simulink model "Complete_scheme_Prove_Balancing"  (R2021a)
settings: Solver=VariableStepAuto  StartTime=0.0  StopTime=60  RelTol=1e-8
PreLoadFcn:
  | data_preload
  | input_preload
values from neighbouring files (symbols this model uses):
  A = [-1/sqrt(2)  1/sqrt(2)     0;      -1/sqrt(6) -1/sqrt(6) sqrt(2/3);       1/sqrt(3)  1/sqrt(3) 1/sqrt(3)]    [data_preload.m]    (also in data_preload_4RW.m = [-a  a  a -a;      -a -a  a  a;       a  a  a  a])
  A_inv = pinv(A)    [data_preload.m]    (also in data_preload_4RW.m)
  A_rw = [-b/J*eye(3) Kt/J*eye(3); -Ke/L*eye(3) -R/L*eye(3)]    [data_preload.m]    (also in data_preload_4RW.m = [-b/J*eye(4) Kt/J*eye(4); -Ke/L*eye(4) -R/L*eye(4)])
  B_rw = [zeros(3); 1/L*eye(3)]    [data_preload.m]    (also in data_preload_4RW.m = [zeros(4); 1/L*eye(4)])
  C_rw = [eye(6); -b/J*eye(3) Kt/J*eye(3)]    [data_preload.m]    (also in data_preload_4RW.m = [eye(8); -b/J*eye(4) Kt/J*eye(4)])
  dt = 0.00001    (= 1e-05)    [RWSizing.m]    (also in data_preload.m = 0.01; data_preload_4RW.m = 0.01)
  G_aug = lqr(A_aug,B_aug,Qlqr,Rlqr)    [data_preload.m]    (also in data_preload_4RW.m)
  G_sim = lqr(A_sim,B_sim,Qlqr,Rlqr)    [data_preload.m]    (also in data_preload_4RW.m)
  I_s = [0.107 0 0; 0 0.108 0; 0 0 0.116]    [data_preload.m]    (also in data_preload_4RW.m)
  I_s_inv = inv(I_s)    [data_preload.m]    (also in data_preload_4RW.m)
  I_w = J*eye(3)    [data_preload.m]    (also in data_preload_4RW.m = J*eye(4))
  I_w_inv = inv(I_w)    [data_preload.m]    (also in data_preload_4RW.m)
  J = 1.74e-4 + 5.1e-7    (= 0.00017451)    [data_preload.m]    (also in data_preload_4RW.m)
  Ke = 0.008    [data_preload.m]    (also in data_preload_4RW.m)
  Kt = 0.00797    [data_preload.m]    (also in data_preload_4RW.m)
  omega = omega*2*pi/60    (= 188.495559215)    [RWSizing.m]    (also in data_preload.m = 250; data_preload_4RW.m = 250)
  vel_slope = theta_tot/(n*t_tot^2*(1-n))    (= 0.0517844942899)    [input_preload.m]
undefined symbols (not defined in the file or in its folder): DiscIntNeverNeededParam
libraries: simulink x28, simulink_extras x14, vrlib x7
settings Model: Creator=gcors  LastModifiedBy=gcors
settings DataIOCC: SaveFormat=Structure

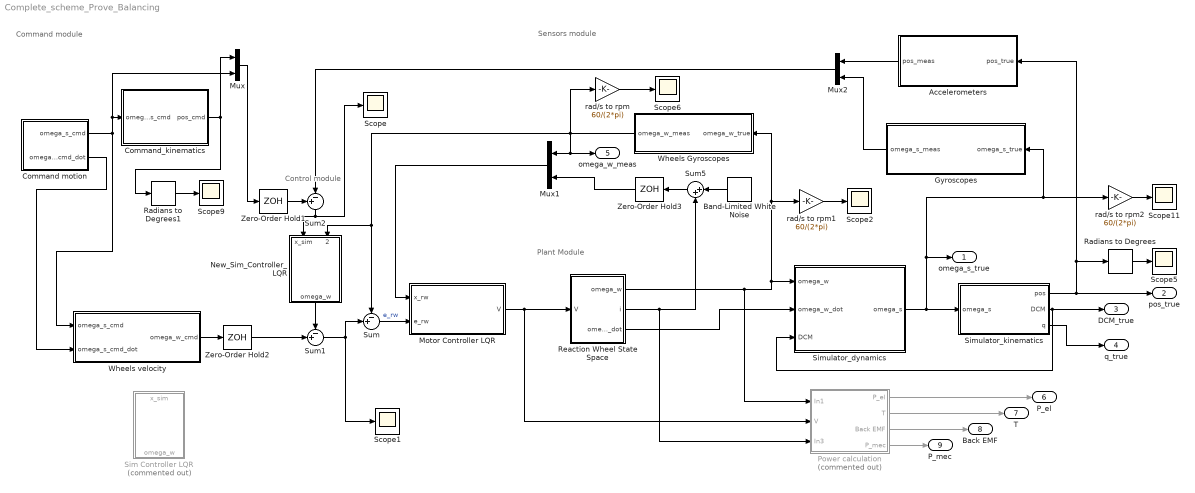
== system Complete_scheme_Prove_Balancing ==
  note: Control module
  note: Sensors module
  note: Plant Module
  note: Command module
  Accelerometers : Subsystem
  Band-Limited White Noise : simulink/Sources/Band-Limited White Noise  Cov=[(0.1^2)/47]  Ts=dt  seed=[23341]
  Command motion : Subsystem
  Command_kinematics : Subsystem
  Gyroscopes : Subsystem
  Motor Controller LQR : Subsystem
  Mux : Mux  Inputs=2
  Mux1 : Mux  Inputs=2
  Mux2 : Mux  Inputs=2
  New_Sim_Controller_LQR : Subsystem
  Power calculation : Subsystem  Commented=on
  Radians to Degrees : simulink_extras/Transformations/Radians to Degrees
  Radians to Degrees1 : simulink_extras/Transformations/Radians to Degrees
  Reaction Wheel State Space : Subsystem
  Scope{,1..2,5..6,9,11} (7 alike) : Scope
  Sim Controller LQR : Subsystem  Commented=on
  Simulator_dynamics : Subsystem
  Simulator_kinematics : Subsystem
  Sum : Sum  Inputs=-+|
  Sum1 : Sum  Inputs=-+|
  Sum2 : Sum  Inputs=+-|
  Sum5 : Sum  Inputs=|++
  Wheels Gyroscopes : Subsystem
  Wheels velocity : Subsystem
  Zero-Order Hold1 : ZeroOrderHold  SampleTime=dt
  Zero-Order Hold2 : ZeroOrderHold  SampleTime=dt
  Zero-Order Hold3 : ZeroOrderHold  SampleTime=dt
  rad/s to rpm : Gain  Gain=60/(2*pi)
  rad/s to rpm1 : Gain  Gain=60/(2*pi)
  rad/s to rpm2 : Gain  Gain=60/(2*pi)
  omega_s_true : Outport  PortDimensions=3
  pos_true : Outport  Port=2  PortDimensions=3
  DCM_true : Outport  Port=3  PortDimensions=[3,3]
  q_true : Outport  Port=4
  omega_w_meas : Outport  Port=5  PortDimensions=3
  P_el : Outport  Port=6
  T : Outport  Port=7
  Back EMF : Outport  Port=8
  P_mec : Outport  Port=9
  wires:
  Simulator_dynamics/1(omega_s) -> rad/s to rpm2/1, Gyroscopes/1(omega_s_true), omega_s_true/1, Simulator_kinematics/1(omega_s)
  Sum/1 -> Motor Controller LQR/2(e_rw)  "e_rw"
  Simulator_kinematics/3(q) -> q_true/1
  Simulator_kinematics/2(DCM) -> Simulator_dynamics/3(DCM), DCM_true/1
  Reaction Wheel State Space/3(omega_w_dot) -> Simulator_dynamics/2(omega_w_dot)
  Radians to Degrees1/1 -> Scope9/1
  Command_kinematics/1(pos_cmd) -> Mux/1, Radians to Degrees1/1
  Command motion/1(omega_s_cmd) -> Mux/2, Command_kinematics/1(omega_s_cmd), Wheels velocity/1(omega_s_cmd)
  Command motion/2(omega_s_cmd_dot) -> Wheels velocity/2(omega_s_cmd_dot)
  Sum1/1 -> Scope1/1, Sum/2
  rad/s to rpm/1 -> Scope6/1
  Reaction Wheel State Space/2(i) -> Sum5/2, Power calculation/3(In3)
  Simulator_kinematics/1(pos) -> Accelerometers/1(pos_true), Radians to Degrees/1, pos_true/1
  Gyroscopes/1(omega_s_meas) -> Mux2/2
  Accelerometers/1(pos_meas) -> Mux2/1
  Mux2/1 -> Sum2/2
  Band-Limited White Noise/1 -> Sum5/1
  Power calculation/1(P_el) -> P_el/1
  Power calculation/2(T) -> T/1
  Power calculation/3(Back EMF) -> Back EMF/1
  Power calculation/4(P_mec) -> P_mec/1
  Mux1/1 -> Motor Controller LQR/1(x_rw)
  Wheels velocity/1(omega_w_cmd) -> Zero-Order Hold2/1
  Mux/1 -> Zero-Order Hold1/1
  Radians to Degrees/1 -> Scope5/1
  Reaction Wheel State Space/1(omega_w) -> Simulator_dynamics/1(omega_w), Wheels Gyroscopes/1(omega_w_true), rad/s to rpm1/1, Power calculation/1(In1)
  Wheels Gyroscopes/1(omega_w_meas) -> rad/s to rpm/1, New_Sim_Controller_LQR/2(omega_w_meas), Sum/1, omega_w_meas/1, Mux1/1
  rad/s to rpm1/1 -> Scope2/1
  Motor Controller LQR/1(V) -> Reaction Wheel State Space/1(V), Power calculation/2(V)
  rad/s to rpm2/1 -> Scope11/1
  Sum5/1 -> Zero-Order Hold3/1
  Zero-Order Hold2/1 -> Sum1/2
  Zero-Order Hold3/1 -> Mux1/2
  Zero-Order Hold1/1 -> Sum2/1
  Sum2/1 -> New_Sim_Controller_LQR/1(x_sim), Scope/1
  New_Sim_Controller_LQR/1(omega_w) -> Sum1/1

== system Complete_scheme_Prove_Balancing/Accelerometers ==
  pos_true : Inport
  Accelerometers model x1 : Subsystem
  Accelerometers model x2 : Subsystem
  Accelerometers model x3 : Subsystem
  Demux2 : Demux  Outputs=3
  Manual Switch : ManualSwitch  CurrentSetting=0
  Mux1 : Mux  Inputs=3
  Zero-Order Hold : ZeroOrderHold  SampleTime=dt
  pos_meas : Outport
  wires:
  Accelerometers model x1/1(pos_xmeas) -> Mux1/1
  Demux2/1 -> Accelerometers model x1/1(pos_x)
  Accelerometers model x2/1(pos_xmeas) -> Mux1/2
  Demux2/2 -> Accelerometers model x2/1(pos_x)
  pos_true/1 -> Manual Switch/1, Demux2/1
  Demux2/3 -> Accelerometers model x3/1(pos_x)
  Accelerometers model x3/1(pos_xmeas) -> Mux1/3
  Mux1/1 -> Manual Switch/2
  Manual Switch/1 -> Zero-Order Hold/1
  Zero-Order Hold/1 -> pos_meas/1

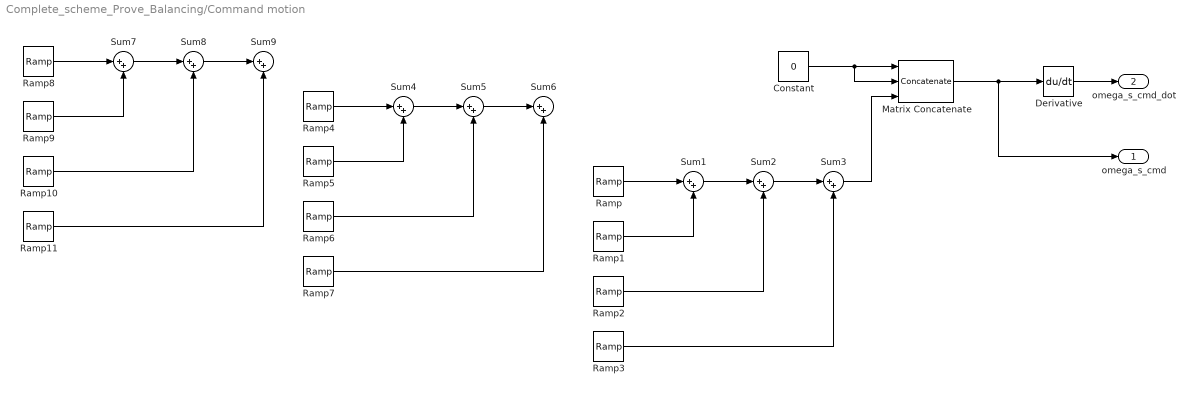
== system Complete_scheme_Prove_Balancing/Command motion ==
  Constant : Constant  Value=0
  Derivative : Derivative
  Matrix Concatenate : Concatenate  NumInputs=3  ConcatenateDimension=2
  Ramp : simulink/Sources/Ramp  slope=vel_slope  start=t0  InitialOutput=0
  Ramp1 : simulink/Sources/Ramp  slope=-vel_slope  start=t1  InitialOutput=0
  Ramp10 : simulink/Sources/Ramp  slope=-0.03  start=52  InitialOutput=0
  Ramp11 : simulink/Sources/Ramp  slope=0.03  start=55  InitialOutput=0
  Ramp2 : simulink/Sources/Ramp  slope=-vel_slope  start=t2  InitialOutput=0
  Ramp3 : simulink/Sources/Ramp  slope=vel_slope  start=t3  InitialOutput=0
  Ramp4 : simulink/Sources/Ramp  slope=0.05  start=30  InitialOutput=0
  Ramp5 : simulink/Sources/Ramp  slope=-0.05  start=33  InitialOutput=0
  Ramp6 : simulink/Sources/Ramp  slope=-0.05  start=37  InitialOutput=0
  Ramp7 : simulink/Sources/Ramp  slope=0.05  start=40  InitialOutput=0
  Ramp8 : simulink/Sources/Ramp  slope=0.03  start=45  InitialOutput=0
  Ramp9 : simulink/Sources/Ramp  slope=-0.03  start=48  InitialOutput=0
  Sum{1..9} (9 alike) : Sum  Inputs=|++
  omega_s_cmd : Outport
  omega_s_cmd_dot : Outport  Port=2
  wires:
  Sum2/1 -> Sum3/1
  Ramp3/1 -> Sum3/2
  Ramp/1 -> Sum1/1
  Ramp1/1 -> Sum1/2
  Ramp2/1 -> Sum2/2
  Sum1/1 -> Sum2/1
  Derivative/1 -> omega_s_cmd_dot/1
  Matrix Concatenate/1 -> Derivative/1, omega_s_cmd/1
  Sum4/1 -> Sum5/1
  Ramp7/1 -> Sum6/2
  Ramp5/1 -> Sum4/2
  Ramp4/1 -> Sum4/1
  Ramp6/1 -> Sum5/2
  Sum5/1 -> Sum6/1
  Sum7/1 -> Sum8/1
  Ramp11/1 -> Sum9/2
  Ramp9/1 -> Sum7/2
  Ramp8/1 -> Sum7/1
  Ramp10/1 -> Sum8/2
  Sum8/1 -> Sum9/1
  Constant/1 -> Matrix Concatenate/1, Matrix Concatenate/2
  Sum3/1 -> Matrix Concatenate/3

== system Complete_scheme_Prove_Balancing/Command_kinematics ==
  omega_s_cmd : Inport  PortDimensions=3
  Euler_angles : MATLAB Function  TreatAsAtomicUnit=on
  Gain : Gain  Gain=1/2
  Integrator1 : Integrator  InitialCondition=[0 0 0 1]'
  Matrix Multiply4 : Product  Multiplication=Matrix(*)
  Normalize Vector : vrlib/Utilities/Normalize Vector  maxzero=0
  OMEGA_matrix : MATLAB Function  TreatAsAtomicUnit=on
  Scope : Scope
  Scope1 : Scope
  getDCM : MATLAB Function  TreatAsAtomicUnit=on
  pos_cmd : Outport  PortDimensions=3
  wires:
  Integrator1/1 -> Normalize Vector/1  "q"
  OMEGA_matrix/1(OMEGA) -> Matrix Multiply4/1
  Gain/1 -> Integrator1/1  "q_dot"
  Matrix Multiply4/1 -> Gain/1
  omega_s_cmd/1 -> OMEGA_matrix/1(omega_s)
  Normalize Vector/1 -> Euler_angles/1(q), Scope/1, Matrix Multiply4/2, getDCM/1(q)
  Euler_angles/1(pos) -> pos_cmd/1
  getDCM/1(DCM) -> Scope1/1

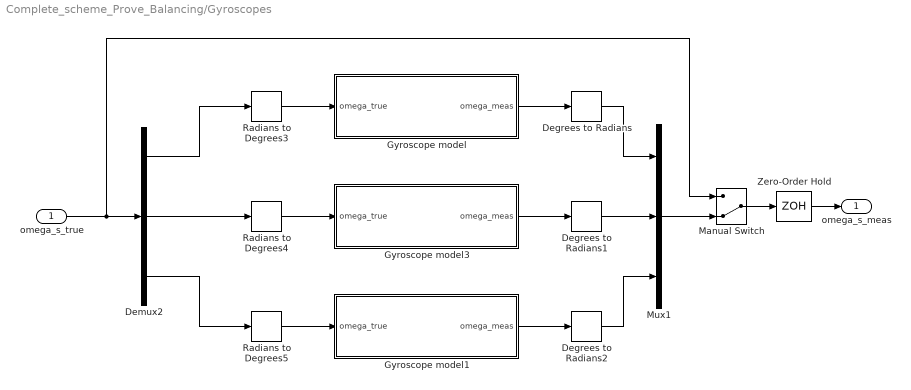
== system Complete_scheme_Prove_Balancing/Gyroscopes ==
  omega_s_true : Inport
  Degrees to Radians : simulink_extras/Transformations/Degrees to Radians
  Degrees to Radians1 : simulink_extras/Transformations/Degrees to Radians
  Degrees to Radians2 : simulink_extras/Transformations/Degrees to Radians
  Demux2 : Demux  Outputs=3
  Gyroscope model : Subsystem
  Gyroscope model1 : Subsystem
  Gyroscope model3 : Subsystem
  Manual Switch : ManualSwitch  CurrentSetting=0
  Mux1 : Mux  Inputs=3
  Radians to Degrees3 : simulink_extras/Transformations/Radians to Degrees
  Radians to Degrees4 : simulink_extras/Transformations/Radians to Degrees
  Radians to Degrees5 : simulink_extras/Transformations/Radians to Degrees
  Zero-Order Hold : ZeroOrderHold  SampleTime=dt
  omega_s_meas : Outport
  wires:
  Gyroscope model3/1(omega_meas) -> Degrees to Radians1/1
  Demux2/2 -> Radians to Degrees4/1
  Degrees to Radians/1 -> Mux1/1
  Demux2/1 -> Radians to Degrees3/1
  Gyroscope model/1(omega_meas) -> Degrees to Radians/1
  Demux2/3 -> Radians to Degrees5/1
  Degrees to Radians1/1 -> Mux1/2
  Radians to Degrees4/1 -> Gyroscope model3/1(omega_true)
  Degrees to Radians2/1 -> Mux1/3
  Radians to Degrees3/1 -> Gyroscope model/1(omega_true)
  Radians to Degrees5/1 -> Gyroscope model1/1(omega_true)
  Gyroscope model1/1(omega_meas) -> Degrees to Radians2/1
  omega_s_true/1 -> Demux2/1, Manual Switch/1
  Mux1/1 -> Manual Switch/2
  Manual Switch/1 -> Zero-Order Hold/1
  Zero-Order Hold/1 -> omega_s_meas/1

== system Complete_scheme_Prove_Balancing/Motor Controller LQR ==
  x_rw : Inport
  e_rw : Inport  Port=2  PortDimensions=3
  Discrete-Time Integrator : DiscreteIntegrator  gainval=1  SampleTime=-1  ICPrevOutput=DiscIntNeverNeededParam  ICPrevScaledInput=DiscIntNeverNeededParam
  G_aug : Constant  Value=G_aug
  Gain : Gain  Gain=-1
  Matrix Multiply : Product  Multiplication=Matrix(*)
  Mux : Mux  Inputs=2
  V : Outport
  wires:
  x_rw/1 -> Mux/1
  Mux/1 -> Matrix Multiply/2
  G_aug/1 -> Matrix Multiply/1
  Matrix Multiply/1 -> Gain/1
  Discrete-Time Integrator/1 -> Mux/2  "x_i"
  Gain/1 -> V/1
  e_rw/1 -> Discrete-Time Integrator/1

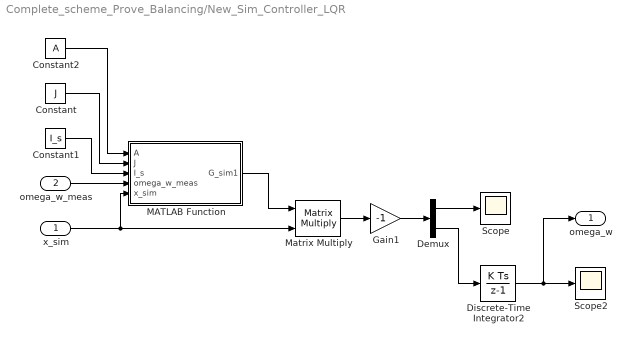
== system Complete_scheme_Prove_Balancing/New_Sim_Controller_LQR ==
  x_sim : Inport
  omega_w_meas : Inport  Port=2
  Constant : Constant  Value=J
  Constant1 : Constant  Value=I_s
  Constant2 : Constant  Value=A
  Demux : Demux  Outputs=2
  Discrete-Time Integrator2 : DiscreteIntegrator  gainval=1  SampleTime=dt  ICPrevOutput=DiscIntNeverNeededParam  ICPrevScaledInput=DiscIntNeverNeededParam
  Gain1 : Gain  Gain=-1
  MATLAB Function : MATLAB Function  TreatAsAtomicUnit=on  SystemSampleTime=dt*10
  Matrix Multiply : Product  Multiplication=Matrix(*)
  Scope : Scope
  Scope2 : Scope
  omega_w : Outport
  wires:
  Matrix Multiply/1 -> Gain1/1
  x_sim/1 -> MATLAB Function/5(x_sim), Matrix Multiply/2
  omega_w_meas/1 -> MATLAB Function/4(omega_w_meas)
  MATLAB Function/1(G_sim1) -> Matrix Multiply/1
  Constant/1 -> MATLAB Function/2(J)
  Constant1/1 -> MATLAB Function/3(I_s)
  Constant2/1 -> MATLAB Function/1(A)
  Discrete-Time Integrator2/1 -> omega_w/1, Scope2/1
  Gain1/1 -> Demux/1
  Demux/2 -> Discrete-Time Integrator2/1
  Demux/1 -> Scope/1

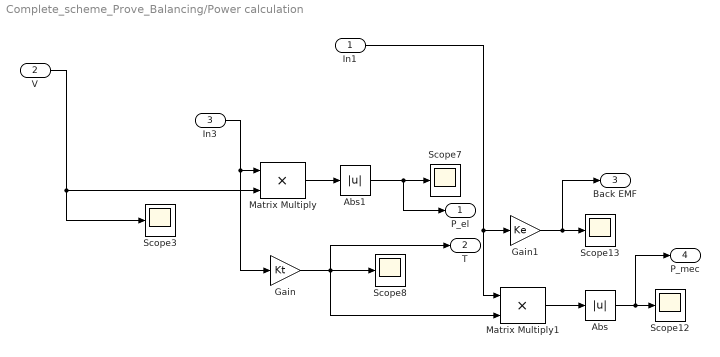
== system Complete_scheme_Prove_Balancing/Power calculation ==
  In1 : Inport
  V : Inport  Port=2
  In3 : Inport  Port=3
  Abs : Abs
  Abs1 : Abs
  Gain : Gain  Gain=Kt
  Gain1 : Gain  Gain=Ke
  Matrix Multiply : Product
  Matrix Multiply1 : Product
  Scope{3,7..8,12..13} (5 alike) : Scope
  P_el : Outport
  T : Outport  Port=2
  Back EMF : Outport  Port=3
  P_mec : Outport  Port=4
  wires:
  Gain/1 -> T/1, Scope8/1, Matrix Multiply1/2
  Matrix Multiply1/1 -> Abs/1
  In1/1 -> Gain1/1, Matrix Multiply1/1
  V/1 -> Matrix Multiply/2, Scope3/1
  Matrix Multiply/1 -> Abs1/1
  Gain1/1 -> Back EMF/1, Scope13/1
  Abs1/1 -> P_el/1, Scope7/1
  Abs/1 -> P_mec/1, Scope12/1
  In3/1 -> Gain/1, Matrix Multiply/1

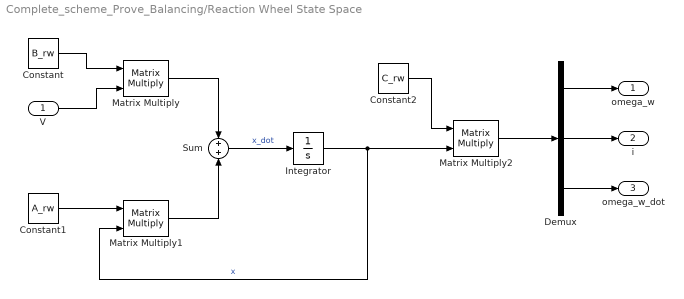
== system Complete_scheme_Prove_Balancing/Reaction Wheel State Space ==
  V : Inport  PortDimensions=3
  Constant : Constant  Value=B_rw
  Constant1 : Constant  Value=A_rw
  Constant2 : Constant  Value=C_rw
  Demux : Demux  Outputs=3
  Integrator : Integrator
  Matrix Multiply : Product  Multiplication=Matrix(*)
  Matrix Multiply1 : Product  Multiplication=Matrix(*)
  Matrix Multiply2 : Product  Multiplication=Matrix(*)
  Sum : Sum  Inputs=+|+
  omega_w : Outport  PortDimensions=3
  i : Outport  Port=2  PortDimensions=3
  omega_w_dot : Outport  Port=3
  wires:
  Integrator/1 -> Matrix Multiply2/2, Matrix Multiply1/2  "x"
  Constant1/1 -> Matrix Multiply1/1
  Matrix Multiply1/1 -> Sum/2
  Constant/1 -> Matrix Multiply/1
  Matrix Multiply/1 -> Sum/1
  Constant2/1 -> Matrix Multiply2/1
  Sum/1 -> Integrator/1  "x_dot"
  Matrix Multiply2/1 -> Demux/1
  Demux/3 -> omega_w_dot/1
  Demux/1 -> omega_w/1
  Demux/2 -> i/1
  V/1 -> Matrix Multiply/2

== system Complete_scheme_Prove_Balancing/Sim Controller LQR ==
  x_sim : Inport
  Discrete-Time Integrator1 : DiscreteIntegrator  gainval=1  SampleTime=dt  ICPrevOutput=DiscIntNeverNeededParam  ICPrevScaledInput=DiscIntNeverNeededParam
  G_sim : Constant  Value=G_sim
  Gain1 : Gain  Gain=-1
  Matrix Multiply : Product  Multiplication=Matrix(*)
  Scope : Scope
  Scope1 : Scope
  omega_w : Outport
  wires:
  G_sim/1 -> Matrix Multiply/1
  Matrix Multiply/1 -> Gain1/1
  x_sim/1 -> Matrix Multiply/2
  Gain1/1 -> Scope/1, Discrete-Time Integrator1/1
  Discrete-Time Integrator1/1 -> Scope1/1, omega_w/1

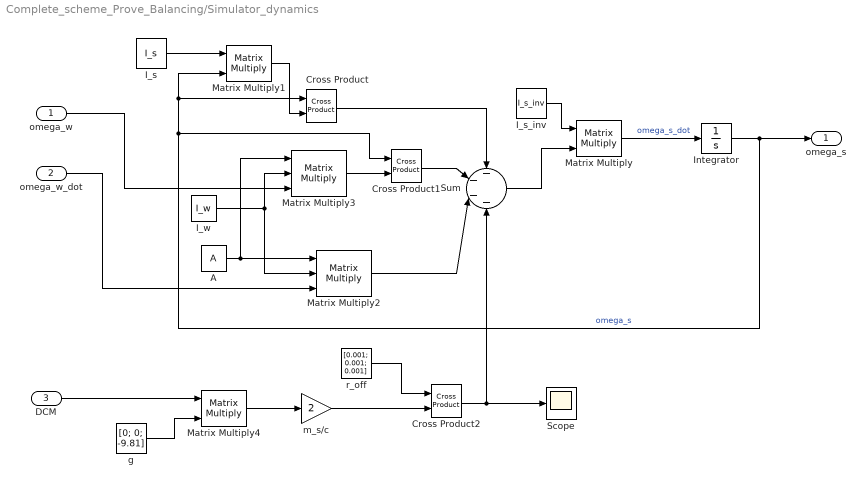
== system Complete_scheme_Prove_Balancing/Simulator_dynamics ==
  omega_w : Inport  PortDimensions=3
  omega_w_dot : Inport  Port=2  PortDimensions=3
  DCM : Inport  Port=3
  A : Constant  Value=A
  Cross Product : vrlib/Utilities/Cross Product
  Cross Product1 : vrlib/Utilities/Cross Product
  Cross Product2 : vrlib/Utilities/Cross Product
  I_s : Constant  Value=I_s
  I_s_inv : Constant  Value=I_s_inv
  I_w : Constant  Value=I_w
  Integrator : Integrator  InitialCondition=[0 0 0]'
  Matrix Multiply : Product  Multiplication=Matrix(*)
  Matrix Multiply1 : Product  Multiplication=Matrix(*)
  Matrix Multiply2 : Product  Inputs=3  Multiplication=Matrix(*)
  Matrix Multiply3 : Product  Inputs=3  Multiplication=Matrix(*)
  Matrix Multiply4 : Product  Multiplication=Matrix(*)
  Scope : Scope
  Sum : Sum  Inputs=----
  g : Constant  Value=[0; 0; -9.81]
  m_s/c : Gain  Gain=2
  r_off : Constant  Value=[0.001; 0.001; 0.001]
  omega_s : Outport  PortDimensions=3
  wires:
  Integrator/1 -> omega_s/1, Cross Product1/1, Cross Product/1, Matrix Multiply1/2  "omega_s"
  Matrix Multiply2/1 -> Sum/3
  I_w/1 -> Matrix Multiply3/2, Matrix Multiply2/2
  A/1 -> Matrix Multiply3/1, Matrix Multiply2/1
  Matrix Multiply3/1 -> Cross Product1/2
  I_s/1 -> Matrix Multiply1/1
  Matrix Multiply/1 -> Integrator/1  "omega_s_dot"
  Sum/1 -> Matrix Multiply/2
  Matrix Multiply1/1 -> Cross Product/2
  Cross Product/1 -> Sum/1
  omega_w/1 -> Matrix Multiply3/3
  Cross Product1/1 -> Sum/2
  omega_w_dot/1 -> Matrix Multiply2/3
  I_s_inv/1 -> Matrix Multiply/1
  DCM/1 -> Matrix Multiply4/1
  g/1 -> Matrix Multiply4/2
  Matrix Multiply4/1 -> m_s/c/1
  m_s/c/1 -> Cross Product2/2
  r_off/1 -> Cross Product2/1
  Cross Product2/1 -> Sum/4, Scope/1

== system Complete_scheme_Prove_Balancing/Simulator_kinematics ==
  omega_s : Inport  PortDimensions=3
  Euler_angles : MATLAB Function  TreatAsAtomicUnit=on
  Gain : Gain  Gain=1/2
  Integrator1 : Integrator  InitialCondition=[0 0 0 1]'
  Matrix Multiply4 : Product  Multiplication=Matrix(*)
  Normalize Vector : vrlib/Utilities/Normalize Vector  maxzero=0
  OMEGA_matrix : MATLAB Function  TreatAsAtomicUnit=on
  getDCM : MATLAB Function  TreatAsAtomicUnit=on
  pos : Outport  PortDimensions=3
  DCM : Outport  Port=2  PortDimensions=[3,3]
  q : Outport  Port=3  PortDimensions=4
  wires:
  Integrator1/1 -> Normalize Vector/1  "q"
  OMEGA_matrix/1(OMEGA) -> Matrix Multiply4/1
  Gain/1 -> Integrator1/1  "q_dot"
  Matrix Multiply4/1 -> Gain/1
  getDCM/1(DCM) -> DCM/1
  omega_s/1 -> OMEGA_matrix/1(omega_s)
  Normalize Vector/1 -> Euler_angles/1(q), q/1, Matrix Multiply4/2, getDCM/1(q)
  Euler_angles/1(pos) -> pos/1

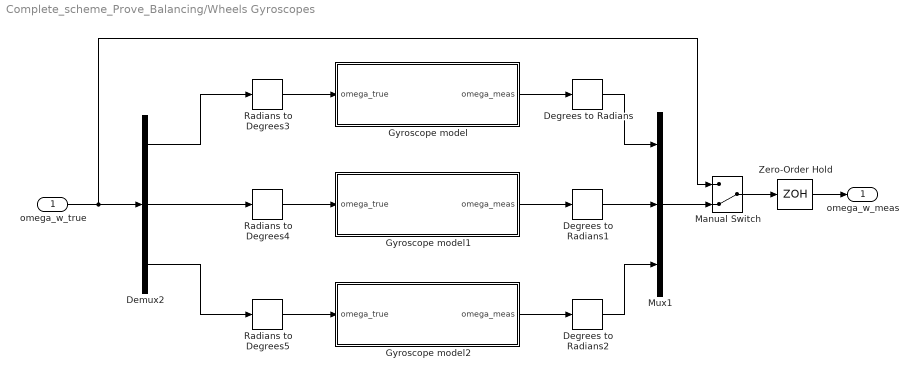
== system Complete_scheme_Prove_Balancing/Wheels Gyroscopes ==
  omega_w_true : Inport
  Degrees to Radians : simulink_extras/Transformations/Degrees to Radians
  Degrees to Radians1 : simulink_extras/Transformations/Degrees to Radians
  Degrees to Radians2 : simulink_extras/Transformations/Degrees to Radians
  Demux2 : Demux  Outputs=3
  Gyroscope model : Subsystem
  Gyroscope model1 : Subsystem
  Gyroscope model2 : Subsystem
  Manual Switch : ManualSwitch  CurrentSetting=0
  Mux1 : Mux  Inputs=3
  Radians to Degrees3 : simulink_extras/Transformations/Radians to Degrees
  Radians to Degrees4 : simulink_extras/Transformations/Radians to Degrees
  Radians to Degrees5 : simulink_extras/Transformations/Radians to Degrees
  Zero-Order Hold : ZeroOrderHold  SampleTime=dt
  omega_w_meas : Outport
  wires:
  Gyroscope model1/1(omega_meas) -> Degrees to Radians1/1
  Demux2/2 -> Radians to Degrees4/1
  Degrees to Radians/1 -> Mux1/1
  Demux2/1 -> Radians to Degrees3/1
  Gyroscope model/1(omega_meas) -> Degrees to Radians/1
  Degrees to Radians1/1 -> Mux1/2
  Radians to Degrees4/1 -> Gyroscope model1/1(omega_true)
  Degrees to Radians2/1 -> Mux1/3
  Radians to Degrees3/1 -> Gyroscope model/1(omega_true)
  Radians to Degrees5/1 -> Gyroscope model2/1(omega_true)
  Gyroscope model2/1(omega_meas) -> Degrees to Radians2/1
  omega_w_true/1 -> Demux2/1, Manual Switch/1
  Mux1/1 -> Manual Switch/2
  Manual Switch/1 -> Zero-Order Hold/1
  Zero-Order Hold/1 -> omega_w_meas/1
  Demux2/3 -> Radians to Degrees5/1

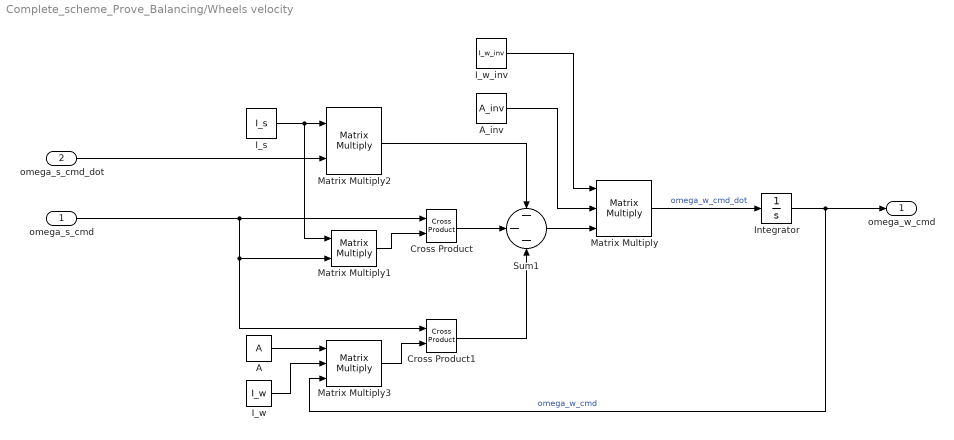
== system Complete_scheme_Prove_Balancing/Wheels velocity ==
  omega_s_cmd : Inport  PortDimensions=3
  omega_s_cmd_dot : Inport  Port=2  PortDimensions=3
  A : Constant  Value=A
  A_inv : Constant  Value=A_inv
  Cross Product : vrlib/Utilities/Cross Product
  Cross Product1 : vrlib/Utilities/Cross Product
  I_s : Constant  Value=I_s
  I_w : Constant  Value=I_w
  I_w_inv : Constant  Value=I_w_inv
  Integrator : Integrator  InitialCondition=[0 0 0]'
  Matrix Multiply : Product  Inputs=3  Multiplication=Matrix(*)
  Matrix Multiply1 : Product  Multiplication=Matrix(*)
  Matrix Multiply2 : Product  Multiplication=Matrix(*)
  Matrix Multiply3 : Product  Inputs=3  Multiplication=Matrix(*)
  Sum1 : Sum  Inputs=---
  omega_w_cmd : Outport  PortDimensions=3
  wires:
  Matrix Multiply/1 -> Integrator/1  "omega_w_cmd_dot"
  A/1 -> Matrix Multiply3/1
  I_s/1 -> Matrix Multiply1/1, Matrix Multiply2/1
  A_inv/1 -> Matrix Multiply/2
  Integrator/1 -> omega_w_cmd/1, Matrix Multiply3/3  "omega_w_cmd"
  omega_s_cmd/1 -> Cross Product/1, Matrix Multiply1/2, Cross Product1/1
  Matrix Multiply1/1 -> Cross Product/2
  Matrix Multiply3/1 -> Cross Product1/2
  omega_s_cmd_dot/1 -> Matrix Multiply2/2
  I_w_inv/1 -> Matrix Multiply/1
  Cross Product1/1 -> Sum1/3
  Cross Product/1 -> Sum1/2
  Sum1/1 -> Matrix Multiply/3
  I_w/1 -> Matrix Multiply3/2
  Matrix Multiply2/1 -> Sum1/1

== system Complete_scheme_Prove_Balancing/Accelerometers/Accelerometers model x1 ==
  pos_x : Inport
  Band-Limited White Noise : simulink/Sources/Band-Limited White Noise  Cov=[(0.00019^2)]  Ts=dt  seed=[23341]
  Floor : Rounding
  Saturation1 : Saturate  UpperLimit=2^13  LowerLimit=-2^13
  Scale factor1 : Gain  Gain=1/1000
  Scale factor3 : Gain  Gain=1000
  Sum7 : Sum  Inputs=|++
  Transfer Fcn2 : TransferFcn  Numerator=[omega^3]  Denominator=[1 2*omega 2*omega^2 omega^3]
  pos_xmeas : Outport
  wires:
  Sum7/1 -> Scale factor3/1
  Scale factor1/1 -> pos_xmeas/1
  Band-Limited White Noise/1 -> Sum7/2
  Floor/1 -> Scale factor1/1
  Transfer Fcn2/1 -> Floor/1
  pos_x/1 -> Sum7/1
  Saturation1/1 -> Transfer Fcn2/1
  Scale factor3/1 -> Saturation1/1

== system Complete_scheme_Prove_Balancing/Accelerometers/Accelerometers model x2 ==
  pos_x : Inport
  Band-Limited White Noise : simulink/Sources/Band-Limited White Noise  Cov=[(0.00019^2)]  Ts=dt  seed=[23341]
  Floor : Rounding
  Saturation1 : Saturate  UpperLimit=2^13  LowerLimit=-2^13
  Scale factor1 : Gain  Gain=1/1000
  Scale factor3 : Gain  Gain=1000
  Sum7 : Sum  Inputs=|++
  Transfer Fcn2 : TransferFcn  Numerator=[omega^3]  Denominator=[1 2*omega 2*omega^2 omega^3]
  pos_xmeas : Outport
  wires:
  Sum7/1 -> Scale factor3/1
  Scale factor1/1 -> pos_xmeas/1
  Band-Limited White Noise/1 -> Sum7/2
  Floor/1 -> Scale factor1/1
  Transfer Fcn2/1 -> Floor/1
  pos_x/1 -> Sum7/1
  Saturation1/1 -> Transfer Fcn2/1
  Scale factor3/1 -> Saturation1/1

== system Complete_scheme_Prove_Balancing/Accelerometers/Accelerometers model x3 ==
  pos_x : Inport
  Band-Limited White Noise : simulink/Sources/Band-Limited White Noise  Cov=[(0.00019^2)]  Ts=dt  seed=[23341]
  Floor : Rounding
  Saturation1 : Saturate  UpperLimit=2^13  LowerLimit=-2^13
  Scale factor1 : Gain  Gain=1/1000
  Scale factor3 : Gain  Gain=1000
  Sum7 : Sum  Inputs=|++
  Transfer Fcn2 : TransferFcn  Numerator=[omega^3]  Denominator=[1 2*omega 2*omega^2 omega^3]
  pos_xmeas : Outport
  wires:
  Sum7/1 -> Scale factor3/1
  Scale factor1/1 -> pos_xmeas/1
  Band-Limited White Noise/1 -> Sum7/2
  Floor/1 -> Scale factor1/1
  Transfer Fcn2/1 -> Floor/1
  pos_x/1 -> Sum7/1
  Saturation1/1 -> Transfer Fcn2/1
  Scale factor3/1 -> Saturation1/1

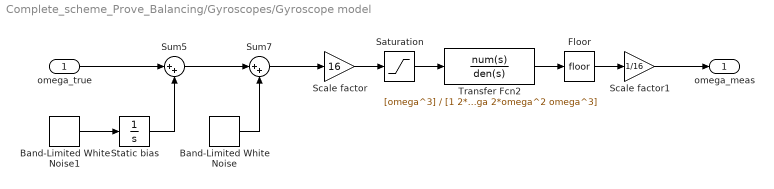
== system Complete_scheme_Prove_Balancing/Gyroscopes/Gyroscope model ==
  omega_true : Inport
  Band-Limited White Noise : simulink/Sources/Band-Limited White Noise  Cov=[(0.3^2)/47]  Ts=dt  seed=[23351]
  Band-Limited White Noise1 : simulink/Sources/Band-Limited White Noise  Cov=[(0.3^2)/47]  Ts=dt  seed=[23351]
  Floor : Rounding
  Saturation : Saturate  UpperLimit=2^15  LowerLimit=-2^15
  Scale factor : Gain  Gain=16
  Scale factor1 : Gain  Gain=1/16
  Static bias : Integrator
  Sum5 : Sum  Inputs=|++
  Sum7 : Sum  Inputs=|++
  Transfer Fcn2 : TransferFcn  Numerator=[omega^3]  Denominator=[1 2*omega 2*omega^2 omega^3]
  omega_meas : Outport
  wires:
  Saturation/1 -> Transfer Fcn2/1
  Scale factor/1 -> Saturation/1
  Sum5/1 -> Sum7/1
  Scale factor1/1 -> omega_meas/1
  Band-Limited White Noise/1 -> Sum7/2
  Static bias/1 -> Sum5/2
  Sum7/1 -> Scale factor/1
  Floor/1 -> Scale factor1/1
  Transfer Fcn2/1 -> Floor/1
  omega_true/1 -> Sum5/1
  Band-Limited White Noise1/1 -> Static bias/1

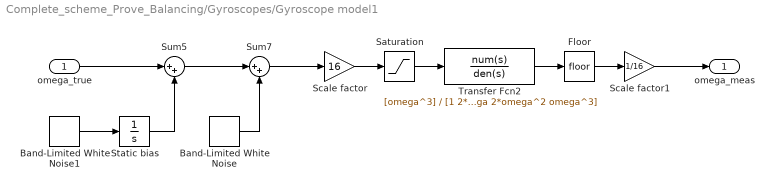
== system Complete_scheme_Prove_Balancing/Gyroscopes/Gyroscope model1 ==
  omega_true : Inport
  Band-Limited White Noise : simulink/Sources/Band-Limited White Noise  Cov=[(0.3^2)/47]  Ts=dt  seed=[23351]
  Band-Limited White Noise1 : simulink/Sources/Band-Limited White Noise  Cov=[(0.3^2)/47]  Ts=dt  seed=[23351]
  Floor : Rounding
  Saturation : Saturate  UpperLimit=2^15  LowerLimit=-2^15
  Scale factor : Gain  Gain=16
  Scale factor1 : Gain  Gain=1/16
  Static bias : Integrator
  Sum5 : Sum  Inputs=|++
  Sum7 : Sum  Inputs=|++
  Transfer Fcn2 : TransferFcn  Numerator=[omega^3]  Denominator=[1 2*omega 2*omega^2 omega^3]
  omega_meas : Outport
  wires:
  Saturation/1 -> Transfer Fcn2/1
  Scale factor/1 -> Saturation/1
  Sum5/1 -> Sum7/1
  Scale factor1/1 -> omega_meas/1
  Band-Limited White Noise/1 -> Sum7/2
  Static bias/1 -> Sum5/2
  Sum7/1 -> Scale factor/1
  Floor/1 -> Scale factor1/1
  Transfer Fcn2/1 -> Floor/1
  omega_true/1 -> Sum5/1
  Band-Limited White Noise1/1 -> Static bias/1

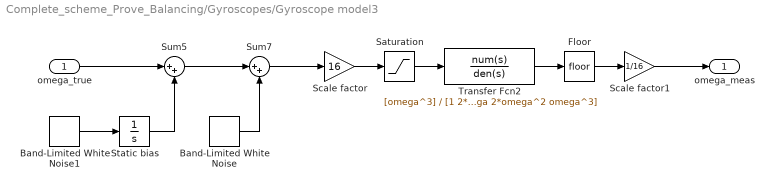
== system Complete_scheme_Prove_Balancing/Gyroscopes/Gyroscope model3 ==
  omega_true : Inport
  Band-Limited White Noise : simulink/Sources/Band-Limited White Noise  Cov=[(0.3^2)/47]  Ts=dt  seed=[23351]
  Band-Limited White Noise1 : simulink/Sources/Band-Limited White Noise  Cov=[(0.3^2)/47]  Ts=dt  seed=[23351]
  Floor : Rounding
  Saturation : Saturate  UpperLimit=2^15  LowerLimit=-2^15
  Scale factor : Gain  Gain=16
  Scale factor1 : Gain  Gain=1/16
  Static bias : Integrator
  Sum5 : Sum  Inputs=|++
  Sum7 : Sum  Inputs=|++
  Transfer Fcn2 : TransferFcn  Numerator=[omega^3]  Denominator=[1 2*omega 2*omega^2 omega^3]
  omega_meas : Outport
  wires:
  Saturation/1 -> Transfer Fcn2/1
  Scale factor/1 -> Saturation/1
  Sum5/1 -> Sum7/1
  Scale factor1/1 -> omega_meas/1
  Band-Limited White Noise/1 -> Sum7/2
  Static bias/1 -> Sum5/2
  Sum7/1 -> Scale factor/1
  Floor/1 -> Scale factor1/1
  Transfer Fcn2/1 -> Floor/1
  omega_true/1 -> Sum5/1
  Band-Limited White Noise1/1 -> Static bias/1

== system Complete_scheme_Prove_Balancing/Wheels Gyroscopes/Gyroscope model ==
  omega_true : Inport
  Band-Limited White Noise : simulink/Sources/Band-Limited White Noise  Cov=[(0.3^2)/47]  Ts=dt  seed=[23341]
  Band-Limited White Noise1 : simulink/Sources/Band-Limited White Noise  Cov=[(0.3^2)/47]  Ts=dt  seed=[23341]
  Floor : Rounding
  Saturation2 : Saturate  UpperLimit=2880000  LowerLimit=-2880000
  Scale factor : Gain  Gain=16
  Scale factor1 : Gain  Gain=1/16
  Static bias : Integrator
  Sum5 : Sum  Inputs=|++
  Sum7 : Sum  Inputs=|++
  Transfer Fcn2 : TransferFcn  Numerator=[omega^3]  Denominator=[1 2*omega 2*omega^2 omega^3]
  omega_meas : Outport
  wires:
  Scale factor/1 -> Saturation2/1
  Sum5/1 -> Sum7/1
  Scale factor1/1 -> omega_meas/1
  Band-Limited White Noise/1 -> Sum7/2
  Static bias/1 -> Sum5/2
  Sum7/1 -> Scale factor/1
  Floor/1 -> Scale factor1/1
  Transfer Fcn2/1 -> Floor/1
  omega_true/1 -> Sum5/1
  Band-Limited White Noise1/1 -> Static bias/1
  Saturation2/1 -> Transfer Fcn2/1

== system Complete_scheme_Prove_Balancing/Wheels Gyroscopes/Gyroscope model1 ==
  omega_true : Inport
  Band-Limited White Noise : simulink/Sources/Band-Limited White Noise  Cov=[(0.3^2)/47]  Ts=dt  seed=[23341]
  Band-Limited White Noise1 : simulink/Sources/Band-Limited White Noise  Cov=[(0.3^2)/47]  Ts=dt  seed=[23341]
  Floor : Rounding
  Saturation2 : Saturate  UpperLimit=2880000  LowerLimit=-2880000
  Scale factor : Gain  Gain=16
  Scale factor1 : Gain  Gain=1/16
  Static bias : Integrator
  Sum5 : Sum  Inputs=|++
  Sum7 : Sum  Inputs=|++
  Transfer Fcn2 : TransferFcn  Numerator=[omega^3]  Denominator=[1 2*omega 2*omega^2 omega^3]
  omega_meas : Outport
  wires:
  Scale factor/1 -> Saturation2/1
  Sum5/1 -> Sum7/1
  Scale factor1/1 -> omega_meas/1
  Band-Limited White Noise/1 -> Sum7/2
  Static bias/1 -> Sum5/2
  Sum7/1 -> Scale factor/1
  Floor/1 -> Scale factor1/1
  Transfer Fcn2/1 -> Floor/1
  omega_true/1 -> Sum5/1
  Band-Limited White Noise1/1 -> Static bias/1
  Saturation2/1 -> Transfer Fcn2/1

== system Complete_scheme_Prove_Balancing/Wheels Gyroscopes/Gyroscope model2 ==
  omega_true : Inport
  Band-Limited White Noise : simulink/Sources/Band-Limited White Noise  Cov=[(0.3^2)/47]  Ts=dt  seed=[23341]
  Band-Limited White Noise1 : simulink/Sources/Band-Limited White Noise  Cov=[(0.3^2)/47]  Ts=dt  seed=[23341]
  Floor : Rounding
  Saturation1 : Saturate  UpperLimit=2880000  LowerLimit=-2880000
  Scale factor : Gain  Gain=16
  Scale factor1 : Gain  Gain=1/16
  Static bias : Integrator
  Sum5 : Sum  Inputs=|++
  Sum7 : Sum  Inputs=|++
  Transfer Fcn2 : TransferFcn  Numerator=[omega^3]  Denominator=[1 2*omega 2*omega^2 omega^3]
  omega_meas : Outport
  wires:
  Scale factor/1 -> Saturation1/1
  Sum5/1 -> Sum7/1
  Scale factor1/1 -> omega_meas/1
  Band-Limited White Noise/1 -> Sum7/2
  Static bias/1 -> Sum5/2
  Sum7/1 -> Scale factor/1
  Floor/1 -> Scale factor1/1
  Transfer Fcn2/1 -> Floor/1
  omega_true/1 -> Sum5/1
  Band-Limited White Noise1/1 -> Static bias/1
  Saturation1/1 -> Transfer Fcn2/1

== matlab function Complete_scheme_Prove_Balancing/Command_kinematics/Euler_angles ==
  data: q input; pos output
function pos = fcn(q)
% function that takes as input the quaternions
% and gives as outputs the Euler angles as
% a vector: pos = [phi theta psi]'

q1 = q(1); q2 = q(2); q3 = q(3); q4 = q(4);

% equations taken from: 
% "Pyramidal reaction wheel arrangement optimization 
% of satellite attitude control subsystem for 
% minimizing power consumption", A.Shirazi, M.Mirshams, 
% Int’l J. of Aeronautical & Space Sci. 15(2), 190–198 (2014) 
phi = atan2( (2*(q1*q4+q2*q3)) , (1-2*(q1^2+q2^2)) );
theta = atan2( 2*(q4*q2-q3*q1),1 );
psi = atan2( (2*(q4*q3+q1*q2)) , (1-2*(q2^2+q3^2)) );

% this is added to have continuity between 0 and 360 deg for psi (yaw)
if q4 < 0
    psi = 2*pi + psi;
end

pos = [phi theta psi]';

end

== matlab function Complete_scheme_Prove_Balancing/Command_kinematics/OMEGA_matrix ==
  data: omega_s input; OMEGA output
function OMEGA = fcn(omega_s)
% function that take as inputs the angular velocity vector omega_s
% and gives as output the skew matrix OMEGA used in the quaternion 
% representation of the kinematics: q_dot = 1/2*OMEGA*q

omega_x = omega_s(1);
omega_y = omega_s(2);
omega_z = omega_s(3);

OMEGA = [   0       omega_z   -omega_y     omega_x;...
         -omega_z      0       omega_x     omega_y;...
          omega_y  -omega_x     0          omega_z;...
         -omega_x  -omega_y   -omega_z         0];
     
end

== matlab function Complete_scheme_Prove_Balancing/Simulator_kinematics/Euler_angles ==
  data: q input; pos output
function pos = fcn(q)
% function that takes as input the quaternions
% and gives as outputs the Euler angles as
% a vector: pos = [phi theta psi]'

q1 = q(1); q2 = q(2); q3 = q(3); q4 = q(4);

% equations taken from: 
% "Pyramidal reaction wheel arrangement optimization 
% of satellite attitude control subsystem for 
% minimizing power consumption", A.Shirazi, M.Mirshams, 
% Int’l J. of Aeronautical & Space Sci. 15(2), 190–198 (2014) 
phi = atan2( (2*(q1*q4+q2*q3)) , (1-2*(q1^2+q2^2)) );
theta = atan2( 2*(q4*q2-q3*q1),1 );
psi = atan2( (2*(q4*q3+q1*q2)) , (1-2*(q2^2+q3^2)) );

% this is added to have continuity between 0 and 360 deg for psi (yaw)
if q4 < 0
    psi = 2*pi + psi;
end

pos = [phi theta psi]';

end

== matlab function Complete_scheme_Prove_Balancing/Simulator_kinematics/OMEGA_matrix ==
  data: omega_s input; OMEGA output
function OMEGA = fcn(omega_s)
% function that take as inputs the angular velocity vector omega_s
% and gives as output the skew matrix OMEGA used in the quaternion 
% representation of the kinematics: q_dot = 1/2*OMEGA*q

omega_x = omega_s(1);
omega_y = omega_s(2);
omega_z = omega_s(3);

OMEGA = [   0       omega_z   -omega_y     omega_x;...
         -omega_z      0       omega_x     omega_y;...
          omega_y  -omega_x     0          omega_z;...
         -omega_x  -omega_y   -omega_z         0];
     
end

== matlab function Complete_scheme_Prove_Balancing/Simulator_kinematics/getDCM ==
  data: q input; DCM output
function DCM = fcn(q)
% function that takes as input the quaternions
% and gives as output the Direction Cosine Matrix DCM

q1 = q(1); q2 = q(2); q3 = q(3); q4 = q(4);

DCM = [q1^2-q2^2-q3^2+q4^2         2*(q1*q2+q3*q4)           2*(q1*q3-q2*q4);...
        2*(q1*q2-q3*q4)         -q1^2+q2^2-q3^2+q4^2         2*(q2*q3+q1*q4);...
        2*(q1*q3+q2*q4)            2*(q2*q3-q1*q4)        -q1^2-q2^2+q3^2+q4^2];

end

== matlab function Complete_scheme_Prove_Balancing/Command_kinematics/getDCM ==
  data: q input; DCM output
function DCM = fcn(q)
% function that takes as input the quaternions
% and gives as output the Direction Cosine Matrix DCM

q1 = q(1); q2 = q(2); q3 = q(3); q4 = q(4);

DCM = [q1^2-q2^2-q3^2+q4^2         2*(q1*q2+q3*q4)           2*(q1*q3-q2*q4);...
        2*(q1*q2-q3*q4)         -q1^2+q2^2-q3^2+q4^2         2*(q2*q3+q1*q4);...
        2*(q1*q3+q2*q4)            2*(q2*q3-q1*q4)        -q1^2-q2^2+q3^2+q4^2];

end

== matlab function Complete_scheme_Prove_Balancing/New_Sim_Controller_LQR/MATLAB Function ==
  data: A input; J input; I_s input; omega_w_meas input; G_sim1 output; x_sim input
function G_sim1 = fcn(A, J, I_s, omega_w_meas, x_sim)
G_sim1 = zeros(6,6);
coder.extrinsic('lqr');


omega_sx = x_sim(4);
omega_sy = x_sim(5);
omega_sz = x_sim(6);

omega_w1 = omega_w_meas(1);
omega_w2 = omega_w_meas(2);
omega_w3 = omega_w_meas(3);

I_sx = I_s(1);
I_sy = I_s(5);
I_sz = I_s(9);

% linearized equations
X1 = 0;
X2 = (1/I_sx) * (-(I_sy-I_sz)*omega_sz - J*(A(3,1)*omega_w1+A(3,2)*omega_w2+A(3,3)*omega_w3));
X3 = (1/I_sx) * (-(I_sy-I_sz)*omega_sy + J*(A(2,1)*omega_w1+A(2,2)*omega_w2+A(2,3)*omega_w3));
X4 = (J/I_sx) * (A(2,1)*omega_sz-A(3,1)*omega_sy);
X5 = (J/I_sx) * (A(2,2)*omega_sz-A(3,2)*omega_sy);
X6 = (J/I_sx) * (A(2,3)*omega_sz-A(3,3)*omega_sy);
X7 = -(J/I_sx) * A(1,1);
X8 = -(J/I_sx) * A(1,2);
X9 = -(J/I_sx) * A(1,3);

Y1 = (1/I_sy) * (-(I_sx-I_sz)*omega_sz + J*(A(3,1)*omega_w1+A(3,2)*omega_w2+A(3,3)*omega_w3));
Y2 = 0;
Y3 = (1/I_sy) * (-(I_sx-I_sz)*omega_sx - J*(A(1,1)*omega_w1+A(1,2)*omega_w2+A(1,3)*omega_w3));
Y4 = (J/I_sy) * (A(3,1)*omega_sx-A(1,1)*omega_sz);
Y5 = (J/I_sy) * (A(3,2)*omega_sx-A(1,2)*omega_sz);
Y6 = (J/I_sy) * (A(3,3)*omega_sx-A(1,3)*omega_sz);
Y7 = -(J/I_sy) * A(2,1);
Y8 = -(J/I_sy) * A(2,2);
Y9 = -(J/I_sy) * A(2,3);

Z1 = (1/I_sz) * (-(I_sy-I_sx)*omega_sy - J*(A(2,1)*omega_w1+A(2,2)*omega_w2+A(2,3)*omega_w3));
Z2 = (1/I_sz) * (-(I_sy-I_sx)*omega_sx + J*(A(1,1)*omega_w1+A(1,2)*omega_w2+A(1,3)*omega_w3));
Z3 = 0;
Z4 = (J/I_sz) * (A(1,1)*omega_sy-A(2,1)*omega_sx);
Z5 = (J/I_sz) * (A(1,2)*omega_sy-A(2,2)*omega_sx);
Z6 = (J/I_sz) * (A(1,3)*omega_sy-A(2,3)*omega_sx);
Z7 = -(J/I_sz) * A(3,1);
Z8 = -(J/I_sz) * A(3,2);
Z9 = -(J/I_sz) * A(3,3);

X = [X1 X2 X3; Y1 Y2 Y3; Z1 Z2 Z3];
Y = [X4 X5 X6; Y4 Y5 Y6; Z4 Z5 Z6];
Z = [X7 X8 X9; Y7 Y8 Y9; Z7 Z8 Z9];


A_sim = [zeros(3) eye(3); zeros(3) X];
B_sim = [zeros(3,6); Y Z];


%---LQR design---
% weighting matrices
q = [1000 1000 1000 100 100 100];
r = [0.1 0.1 0.1 0.01 0.01 0.01];
Qlqr = diag(q);
Rlqr = diag(r);
% LQR gains
% coder.extrinsic('lqr');
G_sim1 = lqr(A_sim,B_sim,Qlqr,Rlqr);

end
